simulink model "convertidor_Buck_simulink"  (R2024b)
settings: Solver=VariableStepAuto  StartTime=0.0  StopTime=0.01  MaxStep=0.01  RelTol=1e-3
InitFcn:
  |     L = 2e-3;    % Inductancia
  |     R = 10;      % Resistencia
  |     C = 10e-6;   % Capacitancia
  |     Uin = 32;   %Voltios
  | 
settings Model: Creator=PC WHALE

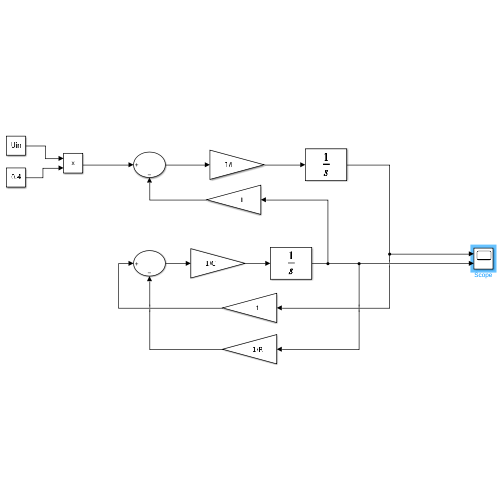
[thumbnail: Simulink's stored preview of the top-level diagram]
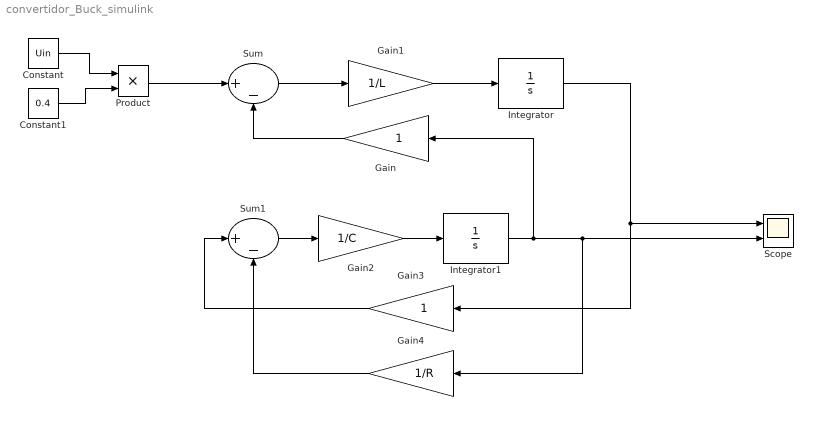
== system convertidor_Buck_simulink ==
  Constant : Constant  Value=Uin
  Constant1 : Constant  Value=0.4
  Gain : Gain
  Gain1 : Gain  Gain=1/L
  Gain2 : Gain  Gain=1/C
  Gain3 : Gain
  Gain4 : Gain  Gain=1/R
  Integrator : Integrator
  Integrator1 : Integrator
  Product : Product
  Scope : Scope  NumInputPorts=2
  Sum : Sum  Inputs=|+-
  Sum1 : Sum  Inputs=|+-
  wires:
  Gain/1 -> Sum/2
  Sum/1 -> Gain1/1
  Gain1/1 -> Integrator/1
  Integrator1/1 -> Scope/2, Gain4/1, Gain/1
  Integrator/1 -> Scope/1, Gain3/1
  Sum1/1 -> Gain2/1
  Gain2/1 -> Integrator1/1
  Gain3/1 -> Sum1/1
  Gain4/1 -> Sum1/2
  Constant/1 -> Product/1
  Constant1/1 -> Product/2
  Product/1 -> Sum/1
